simulink library "sf_mask_lib"  (R2017b)
settings: Solver=ode45  StartTime=0.0  StopTime=10.0  RelTol=1e-3  EnableMultiTasking=on
settings Model: Creator=The MathWorks, Inc.  LastModifiedBy=The MathWorks, Inc.
settings DataIOCC: LimitDataPoints=on  SaveFormat=Array
settings OptimizationCC: ExpressionDepthLimit=2147483647  LifeSpan=inf
settings DebuggingCC: UnderspecifiedInitializationDetection=Classic  MergeDetectMultiDrivingBlocksExec=none  SolverPrmCheckMsg=warning  StateNameClashWarn=warning  SFUnexpectedBacktrackingDiag=warning  SFNoUnconditionalDefaultTransitionDiag=warning  SFExecutionAtInitializationDiag=none
settings HardwareCC: ProdBitPerPointer=32  ProdBitPerSizeT=32  ProdBitPerPtrDiffT=32  ProdLargestAtomicFloat=None  ProdIntDivRoundTo=Undefined  ProdEndianess=Unspecified  ProdWordSize=32  ProdHWDeviceType=32-bit Generic
settings ModelReferenceCC: PropagateSignalLabelsOutOfModel=off
settings CodeAppCC: StateflowObjectComments=on
settings GRTTargetCC: TargetLangStandard=C89/C90 (ANSI)  GeneratePreprocessorConditionals=Disable all
settings ConfigComp: CovMetricSettings=dw  CovHtmlReporting=on  CovSaveCumulativeToWorkspaceVar=on  CovSaveSingleToWorkspaceVar=on  CovExternalEMLEnable=off

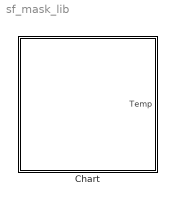
== system sf_mask_lib ==
  Chart : Stateflow chart  TreatAsAtomicUnit=on  mask{AmbTemp=85, DesiredTemp=70, btuSetting=20000}
      mask prompts: AmbTemp "Ambient Temperature"; DesiredTemp "Desired Temperature"; btuSetting "AC Power"
      mask init:
      | if btuSetting == 1
      |     btuValue = 10000;
      | elseif btuSetting == 2
      |     btuValue = 20000;
      | end

== stateflow chart sf_mask_lib/Chart ==
  state AC_OFF
    en,du:Temp = Temp + 0.05*(AmbTemp - Temp);
  state AC_ON
    en,du:Temp = Temp - btuValue/20000;
  (default) -> AC_OFF : {Temp = AmbTemp;}
  AC_OFF -> AC_ON : [Temp >= DesiredTemp]
  AC_ON -> AC_OFF : [Temp < DesiredTemp]
  data: AmbTemp parameter; DesiredTemp parameter; Temp output double; btuValue parameter
